simulink model "test_simulink_sym_block"  (R2022b)
settings: Solver=VariableStepAuto  StartTime=0.0  StopTime=10.0  RelTol=1e-3
settings Model: Creator=ge26jow  LastModifiedBy=ge26jow

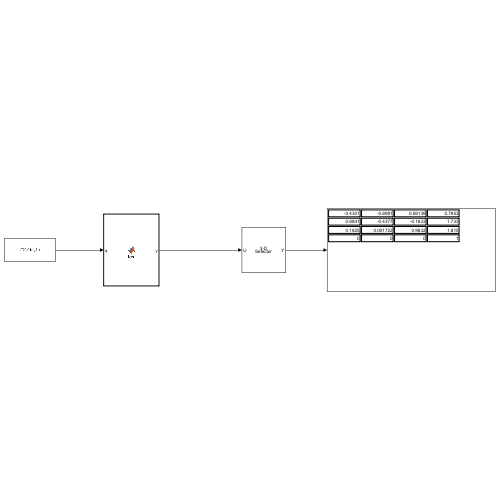
[thumbnail: Simulink's stored preview of the top-level diagram]
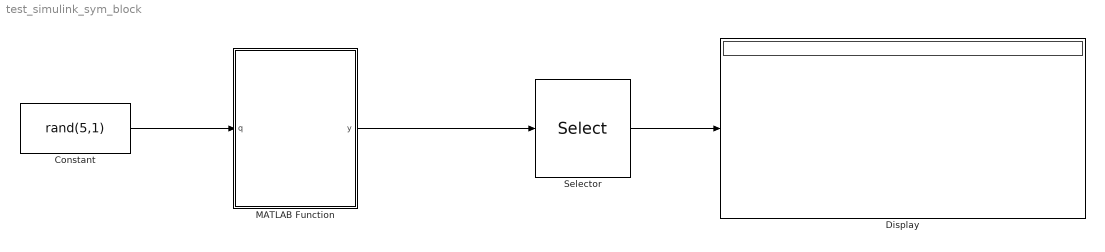
== system test_simulink_sym_block ==
  Constant : Constant  Value=rand(5,1)
  Display : Display
  MATLAB Function : MATLAB Function  TreatAsAtomicUnit=on
  Selector : Selector  NumberOfDimensions=3  InputPortWidth=3  IndexOptions=Index vector (dialog),Index vector (dialog),Index vector (dialog)  Indices=[1:4],[1:4],[4]  OutputSizes=1,1,1
  wires:
  Constant/1 -> MATLAB Function/1(q)
  MATLAB Function/1(y) -> Selector/1
  Selector/1 -> Display/1

== matlab function test_simulink_sym_block/MATLAB Function ==
  data: q input; y output
function y = fcn(q)
w_T_all_sym = T_all_links_from_q_finger_example(q(:));
y = w_T_all_sym;
